simulink model "V3_AusgleichsPolynomPsi__d"  (R2016a)
settings: Solver=FixedStepDiscrete  StartTime=0.0  StopTime=10  FixedStep=0.02  RelTol=1e-3
StopFcn:
  | V3_AusgleichsPolynomPsi__d_terminate
undefined symbols (not defined in the file or in its folder): rpm, rpm_factor
settings Model: SimulationMode=external  ExtModeTrigDuration=1500  Creator=ich  LastModifiedBy=ich
settings OptimizationCC: OptimizeModelRefInitCode=on  LifeSpan=1  MaxStackSize=64
settings HardwareCC: ProdBitPerPointer=32  ProdLargestAtomicInteger=Long  ProdLargestAtomicFloat=Double  ProdWordSize=32  ProdHWDeviceType=ARM Compatible->ARM Cortex
settings RTWCC: SystemTargetFile=ert.tlc  HardwareBoard=STM32F4-Discovery  TemplateMakefile=ert_default_tmf  GenerateReport=on  CustomInclude=MotorBlock\include  Toolchain=GNU Tools for ARM Embedded Processors  IncludeHyperlinkInReport=on  LaunchReport=on  GenerateTraceInfo=on  GenerateTraceReport=on  GenerateTraceReportSl=on  GenerateTraceReportSf=on  GenerateTraceReportEml=on
settings RTWCC: CustomSource=|
  | MotorBlock\source\ADC.c
  | MotorBlock\source\stm32f4xx_adc.c
  | MotorBlock\source\stm32f4xx_tim.c
  | MotorBlock\source\MotorControl.c
  | MotorBlock\Motor_wrapper.c
settings CodeAppCC: ForceParamTrailComments=on  IgnoreCustomStorageClasses=off  OperatorAnnotations=on  SimulinkDataObjDesc=on  SFDataObjDesc=on  MATLABFcnDesc=on  InsertBlockDesc=on  MATLABSourceComments=on

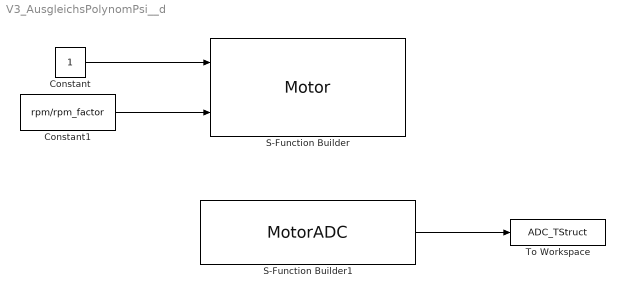
== system V3_AusgleichsPolynomPsi__d ==
  Constant : Constant  OutDataTypeStr=Inherit: Inherit via back propagation
  Constant1 : Constant  Value=rpm/rpm_factor  OutDataTypeStr=single
  S-Function Builder : S-Function  InitFcn=try, set_param(gcb,'FunctionName','Motor'), end  FunctionName=Motor  SFunctionModules=Motor_wrapper  SFunctionDeploymentMode=off  EnableBusSupport=off  mask(S-Function Builder){}
      mask help: Simulink:masks:SFunctionBuilder_MD
      mask init:
      | val = [[.9  0.75 0.75 1 1 .9 .9 1]',[1 1 0.75 0.75 .9 .9 1 .9]'];try , sys = get_param(gcb,'SfunBuilderFcnName');if isempty(sys), sys = get_param(gcb,'FunctionName'); end,catch, sys = get_param(gcb,'FunctionName'); end
      settings: CopyFcn=set_param(gcbh,'LinkStatus','none')  PreSaveFcn=try, set_param(gcb,'FunctionName','Motor'), end  OpenFcn=sfunctionwizard(gcbh)
      mask Display: plot(val(:,1),val(:,2)),disp(sys), port_label('input',1,'EnableState'), port_label('input',2,'Torque')
  S-Function Builder1 : S-Function  InitFcn=try, set_param(gcb,'FunctionName','MotorADC'), end  FunctionName=MotorADC  SFunctionModules=MotorADC_wrapper  SFunctionDeploymentMode=off  EnableBusSupport=off  mask(S-Function Builder){}
      mask help: Simulink:masks:SFunctionBuilder_MD
      mask init: same as V3_AusgleichsPolynomPsi__d/S-Function Builder
      settings: CopyFcn=set_param(gcbh,'LinkStatus','none')  PreSaveFcn=try, set_param(gcb,'FunctionName','MotorADC'), end  OpenFcn=sfunctionwizard(gcbh)
      mask Display: plot(val(:,1),val(:,2)),disp(sys), port_label('output',1,'MotorADC')
  To Workspace : ToWorkspace  VariableName=ADC_TStruct  SaveFormat=Structure With Time  SampleTime=-1
  wires:
  Constant/1 -> S-Function Builder/1
  Constant1/1 -> S-Function Builder/2
  S-Function Builder1/1 -> To Workspace/1
